simulink model "CalculatorRoot"  (R2014b)
settings: Solver=ode45  StartTime=0.0  StopTime=10.0  RelTol=1e-3
PreLoadFcn:
  | addpath('../Divide');
  | addpath('../CommonLibraries');
  | addpath('../ProcAbs');
  | addpath('../ProcAdd');
  | addpath('../Utilities');
settings Model: Creator=PLM\yymatlab  LastModifiedBy=patankar
settings DataIOCC: SignalLoggingSaveFormat=ModelDataLogs
settings OptimizationCC: ExpressionDepthLimit=2147483647
settings DebuggingCC: UnderspecifiedInitializationDetection=Classic  MergeDetectMultiDrivingBlocksExec=none  FcnCallInpInsideContextMsg=EnableAllAsWarning  FrameProcessingCompatibilityMsg=error  StateNameClashWarn=warning
settings GRTTargetCC: CombineOutputUpdateFcns=off  GRTInterface=on
settings ConfigComp: CovMetricSettings=dw  CovHtmlReporting=on  CovSaveCumulativeToWorkspaceVar=on  CovSaveSingleToWorkspaceVar=on  CovModelRefEnable=Off  CovExternalEMLEnable=off  CovSFcnEnable=off

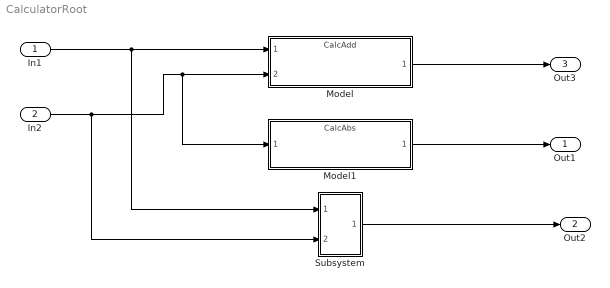
== system CalculatorRoot ==
  In1 : Inport
  In2 : Inport  Port=2
  Model : ModelReference  ModelNameDialog=CalcAdd  SimulationMode=Normal  ModelReferenceVersion=1.5  CopyOfModelName=CalcAdd  DefaultDataLogging=on
  Model1 : ModelReference  ModelNameDialog=CalcAbs  SimulationMode=Normal  ModelReferenceVersion=1.4  CopyOfModelName=CalcAbs  DefaultDataLogging=on
  Subsystem : Subsystem
  Out1 : Outport
  Out2 : Outport  Port=2
  Out3 : Outport  Port=3
  wires:
  In1/1 -> Subsystem/1(In1), Model/1
  In2/1 -> Subsystem/2(In2), Model1/1, Model/2
  Model/1 -> Out3/1
  Model1/1 -> Out1/1
  Subsystem/1(Out1) -> Out2/1

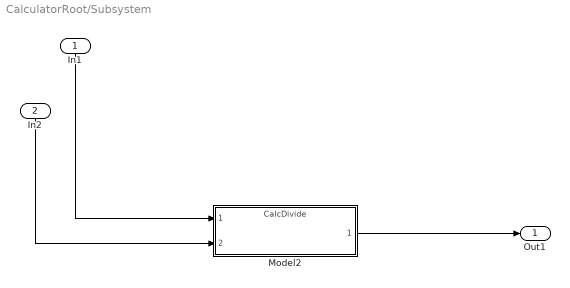
== system CalculatorRoot/Subsystem ==
  In1 : Inport
  In2 : Inport  Port=2
  Model2 : ModelReference  ModelNameDialog=CalcDivide  SimulationMode=Normal  ModelReferenceVersion=1.7  CopyOfModelName=CalcDivide  DefaultDataLogging=on
  Out1 : Outport
  wires:
  Model2/1 -> Out1/1
  In1/1 -> Model2/1
  In2/1 -> Model2/2
